simulink model "teleoperation_simscape"  (R2018a)
settings: Solver=ode45  StartTime=0.0  StopTime=10  RelTol=1e-3
values from neighbouring files (symbols this model uses):
  B_e = 0.01    [simulinkTeleop.m]
  B_h = humanDamp*armL    (= 0.4)    [simulinkTeleop.m]
  B_v = 0.15    [simulinkTeleop.m]
  J_m = 0.0005    [simulinkTeleop.m]
  J_s = 0.0005    [simulinkTeleop.m]
  J_v = 0.0    (= 0)    [simulinkTeleop.m]
  K_e = 1000    [simulinkTeleop.m]
  K_h = humanStiff*armL    (= 20)    [simulinkTeleop.m]
  K_v = 100.0    (= 100)    [simulinkTeleop.m]
  theta_s_contact = -0.0    (= 0)    [simulinkTeleop.m]
undefined symbols (not defined in the file or in its folder): X, Y, Z
libraries: sm_lib x14, cstblocks x5, nesl_utility x3, simulink x1
settings Model: Creator=dinies33  LastModifiedBy=giuseppe

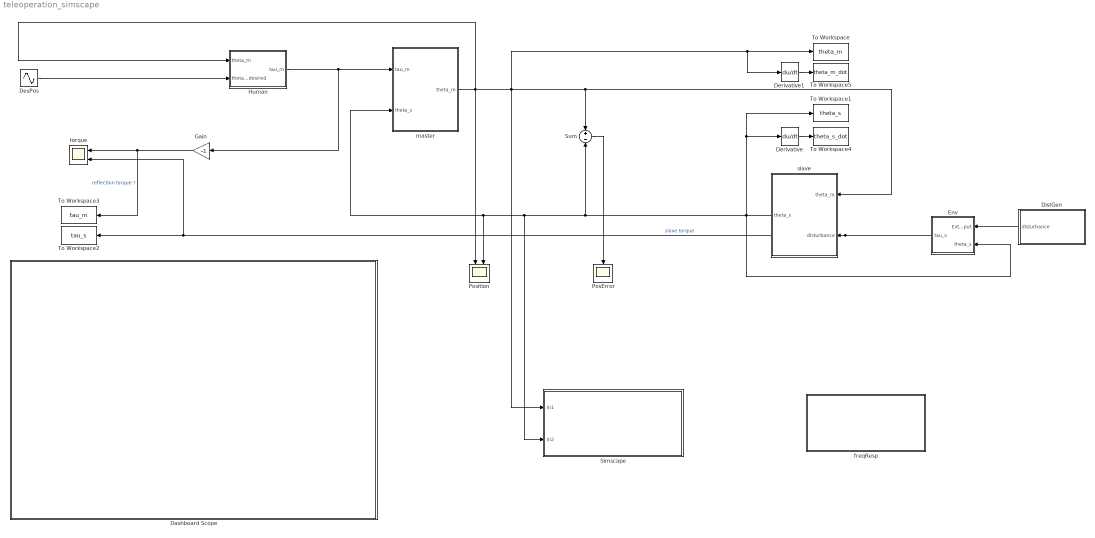
== system teleoperation_simscape ==
  Dashboard Scope : Subsystem  DialogController=hmiCreateDDGDialog  IsWebBlock=on  mask(MWDashboardBlock){webBlockId=d953983e-eab8-4310-ba24-9145e9f5b59c, webBlockType=sdiscope, ShowInitialText=on, HMISrcModelName=teleoperation_simscape}
      mask prompts: webBlockId "WebBlock Id"; webBlockType "WebBlock Type"; HMISrcModelName "Source Model"
      mask help: SimulinkHMI:dialogs:HMIScopeDialogDesc
      mask Help: helpview([docroot '/mapfiles/simulink.map'], 'hmi_scope')
      mask Display:
      | if strcmp(get_param(bdroot(gcb),'BlockDiagramType'), 'library')
      |     image([(matlabroot) '/toolbox/simulink/hmi/icons/DashboardScope.png']);
      | end
  Derivative : Derivative  CoefficientInTFapproximation=0
  Derivative1 : Derivative  CoefficientInTFapproximation=0
  DesPos : Sin  Amplitude=0.18  Frequency=0.11*(6.28)  SampleTime=0
  DistGen : Subsystem
  Env : Subsystem
  Gain : Gain  Gain=-1
  Human : Subsystem
  PosError : Scope
  Position : Scope  NumInputPorts=2
  Simscape : Subsystem
  Sum : Sum  Inputs=+-
  To Workspace : ToWorkspace  VariableName=theta_m  SampleTime=-1
  To Workspace1 : ToWorkspace  VariableName=theta_s  SampleTime=-1
  To Workspace2 : ToWorkspace  VariableName=tau_s  SampleTime=-1
  To Workspace3 : ToWorkspace  VariableName=tau_m  SampleTime=-1
  To Workspace4 : ToWorkspace  VariableName=theta_s_dot  SampleTime=-1
  To Workspace5 : ToWorkspace  VariableName=theta_m_dot  SampleTime=-1
  freqResp : Subsystem
  master : Subsystem
  "slave " : Subsystem
  torque : Scope  NumInputPorts=2
  wires:
  Env/1("tau_s ") -> torque/2, To Workspace2/1, "slave "/2(disturbance)  "slave torque"
  DesPos/1 -> Human/2(theta_desired)
  master/1(theta_m) -> Sum/1, "slave "/1("theta_m "), Derivative1/1, To Workspace/1, Simscape/1(In1), Human/1(theta_m), Position/1
  Human/1(tau_m) -> Gain/1, master/1(tau_m)
  "slave "/1(theta_s) -> Derivative/1, To Workspace1/1, Sum/2, Simscape/2(In2), master/2(theta_s), Position/2, Env/2(theta_s)
  Gain/1 -> To Workspace3/1, torque/1  "reflection torque ?"
  Sum/1 -> PosError/1
  Derivative1/1 -> To Workspace5/1
  Derivative/1 -> To Workspace4/1
  DistGen/1(disturbance) -> Env/1(External_input)

== system teleoperation_simscape/Dashboard Scope ==

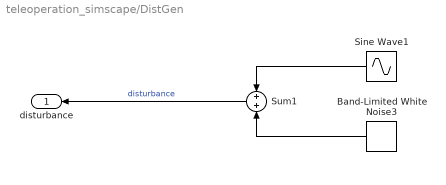
== system teleoperation_simscape/DistGen ==
  Band-Limited White Noise3 : simulink/Sources/Band-Limited White Noise  Cov=0.001  Ts=1/20  seed=[12345]
  Sine Wave1 : Sin  Amplitude=0.015  Frequency=20*(6.28)  SampleTime=0
  Sum1 : Sum
  disturbance : Outport
  wires:
  Band-Limited White Noise3/1 -> Sum1/2
  Sum1/1 -> disturbance/1  "disturbance"
  Sine Wave1/1 -> Sum1/1

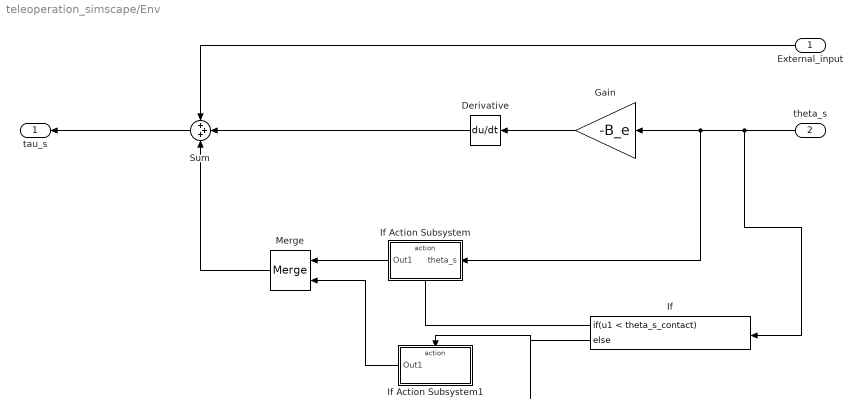
== system teleoperation_simscape/Env ==
  External_input : Inport
  theta_s : Inport  Port=2
  Derivative : Derivative  CoefficientInTFapproximation=0
  Gain : Gain  Gain=-B_e
  If : If  IfExpression=u1 < theta_s_contact
  If Action Subsystem : Subsystem  TreatAsAtomicUnit=on
  If Action Subsystem1 : Subsystem  TreatAsAtomicUnit=on
  Merge : Merge
  Sum : Sum  Inputs=+++
  "tau_s " : Outport
  wires:
  External_input/1 -> Sum/1
  theta_s/1 -> If/1, If Action Subsystem/1(theta_s), Gain/1
  Gain/1 -> Derivative/1
  Derivative/1 -> Sum/2
  Sum/1 -> "tau_s "/1
  If/2 -> If Action Subsystem1/Action
  If/1 -> If Action Subsystem/Action
  If Action Subsystem1/1(Out1) -> Merge/2
  If Action Subsystem/1(Out1) -> Merge/1
  Merge/1 -> Sum/3

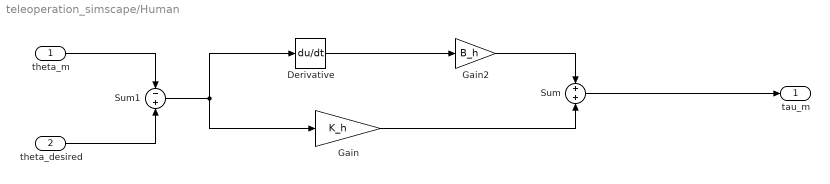
== system teleoperation_simscape/Human ==
  theta_m : Inport
  theta_desired : Inport  Port=2
  Derivative : Derivative  CoefficientInTFapproximation=0
  Gain : Gain  Gain=K_h
  Gain2 : Gain  Gain=B_h
  Sum : Sum  Inputs=+|+
  Sum1 : Sum  Inputs=-|+
  tau_m : Outport
  wires:
  Derivative/1 -> Gain2/1
  theta_m/1 -> Sum1/1
  theta_desired/1 -> Sum1/2
  Sum1/1 -> Derivative/1, Gain/1
  Gain2/1 -> Sum/1
  Gain/1 -> Sum/2
  Sum/1 -> tau_m/1

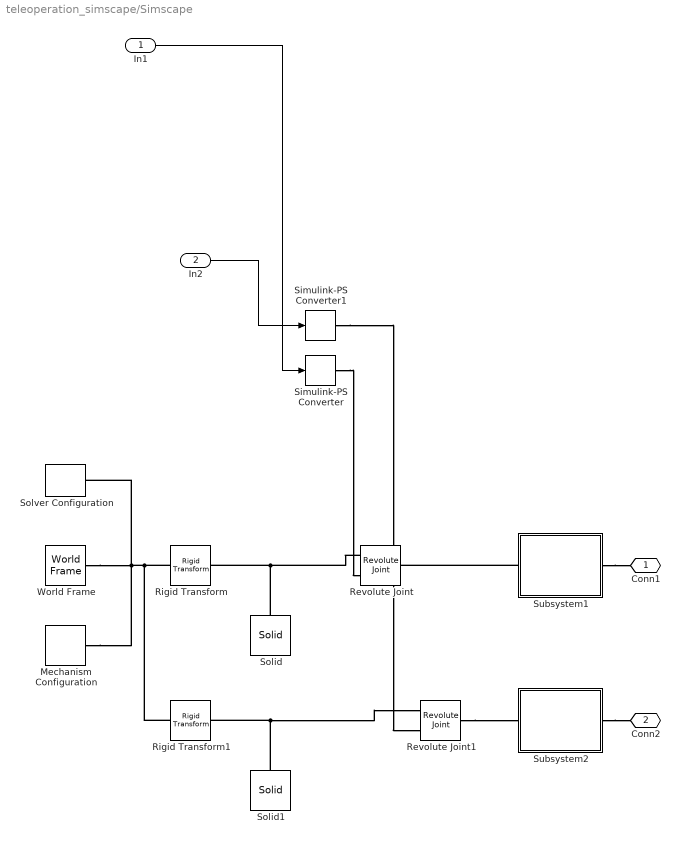
== system teleoperation_simscape/Simscape ==
  In1 : Inport
  In2 : Inport  Port=2
  Mechanism Configuration : sm_lib/Utilities/Mechanism Configuration  UniformGravity=Constant  GravityVector=[0 -9.81 0]  GravityUnits=m/s^2  LinearizationDelta=0.001
  Revolute Joint : sm_lib/Joints/Revolute Joint  SenseConstraintForce=off  SenseConstraintForceX=off  SenseConstraintForceY=off  SenseConstraintForceZ=off  SenseConstraintTorque=off  SenseConstraintTorqueX=off  SenseConstraintTorqueY=off  SenseConstraintTorqueZ=off  SenseTotalForce=off  SenseTotalForceX=off  SenseTotalForceY=off  SenseTotalForceZ=off  SenseTotalTorque=off  SenseTotalTorqueX=off  SenseTotalTorqueY=off  SenseTotalTorqueZ=off  CompositeWrenchDir=FollowerOnBase  CompositeWrenchFrame=BaseFrame  EquilibriumPosition=0  EquilibriumPositionUnits=deg  SpringStiffness=0  SpringStiffnessUnits=N*m/deg  DampingCoefficient=0  DampingCoefficientUnits=N*m/(deg/s)  TorqueActuationMode=ComputedTorque  MotionActuationMode=InputMotion  SensePosition=off  SenseVelocity=off  SenseAcceleration=off  SenseTorqueForce=off  PositionTargetSpecify=off  PositionTargetPriority=High  PositionTargetValue=0  PositionTargetValueUnits=deg  VelocityTargetSpecify=off  VelocityTargetPriority=High  VelocityTargetValue=0  VelocityTargetValueUnits=deg/s
  Revolute Joint1 : sm_lib/Joints/Revolute Joint  SenseConstraintForce=off  SenseConstraintForceX=off  SenseConstraintForceY=off  SenseConstraintForceZ=off  SenseConstraintTorque=off  SenseConstraintTorqueX=off  SenseConstraintTorqueY=off  SenseConstraintTorqueZ=off  SenseTotalForce=off  SenseTotalForceX=off  SenseTotalForceY=off  SenseTotalForceZ=off  SenseTotalTorque=off  SenseTotalTorqueX=off  SenseTotalTorqueY=off  SenseTotalTorqueZ=off  CompositeWrenchDir=FollowerOnBase  CompositeWrenchFrame=BaseFrame  EquilibriumPosition=0  EquilibriumPositionUnits=deg  SpringStiffness=0  SpringStiffnessUnits=N*m/deg  DampingCoefficient=0  DampingCoefficientUnits=N*m/(deg/s)  TorqueActuationMode=ComputedTorque  MotionActuationMode=InputMotion  SensePosition=off  SenseVelocity=off  SenseAcceleration=off  SenseTorqueForce=off  PositionTargetSpecify=off  PositionTargetPriority=High  PositionTargetValue=0  PositionTargetValueUnits=deg  VelocityTargetSpecify=off  VelocityTargetPriority=High  VelocityTargetValue=0  VelocityTargetValueUnits=deg/s
  Rigid Transform : sm_lib/Frames and Transforms/Rigid Transform  TranslationMethod=StandardAxis  TranslationStandardOffset=-0.2  TranslationLengthUnit=m  TranslationStandardAxis=+X  TranslationCartesianOffset=[0 0 0]  TranslationROffset=0  TranslationROffsetUnits=m  TranslationZOffset=0  TranslationZOffsetUnits=m  TranslationThetaOffset=0  TranslationThetaOffsetUnits=deg  RotationMethod=StandardAxis  RotationAngleUnits=deg  RotationStandardAxis=+Z  RotationAngle=-90  RotationArbitraryAxis=[0 0 1]  FollAlignAxisA=+X  BaseAlignAxisA=+Y  FollAlignAxisB=+Y  BaseAlignAxisB=+Z  RotationSequenceAxes=FollowerAxes  RotationSequence=XYX  RotationSequenceAngles=[0 0 0]  RotationSequenceAnglesUnits=deg  RotationMatrix=[1 0 0; 0 1 0; 0 0 1]
  Rigid Transform1 : sm_lib/Frames and Transforms/Rigid Transform  TranslationMethod=StandardAxis  TranslationStandardOffset=0.2  TranslationLengthUnit=m  TranslationStandardAxis=+X  TranslationCartesianOffset=[0 0 0]  TranslationROffset=0  TranslationROffsetUnits=m  TranslationZOffset=0  TranslationZOffsetUnits=m  TranslationThetaOffset=0  TranslationThetaOffsetUnits=deg  RotationMethod=StandardAxis  RotationAngleUnits=deg  RotationStandardAxis=+Z  RotationAngle=-90  RotationArbitraryAxis=[0 0 1]  FollAlignAxisA=+X  BaseAlignAxisA=+Y  FollAlignAxisB=+Y  BaseAlignAxisB=+Z  RotationSequenceAxes=FollowerAxes  RotationSequence=XYX  RotationSequenceAngles=[0 0 0]  RotationSequenceAnglesUnits=deg  RotationMatrix=[1 0 0; 0 1 0; 0 0 1]
  Simulink-PS Converter : nesl_utility/Simulink-PS Converter  PhysicalDomain=network_engine_domain  SubClassName=ps_input  LeftPortType=input  RightPortType=output  PseudoPeriodic=off  Frequencies=[]  NoiseDistribution=none  NoiseParameters=[]  Unit=rad  AffineConversion=on  FilteringAndDerivatives=filter  SimscapeFilterOrder=2  InputFilterTimeConstant=0.001  UdotUserProvided=0
  Simulink-PS Converter1 : nesl_utility/Simulink-PS Converter  PhysicalDomain=network_engine_domain  SubClassName=ps_input  LeftPortType=input  RightPortType=output  PseudoPeriodic=off  Frequencies=[]  NoiseDistribution=none  NoiseParameters=[]  Unit=rad  AffineConversion=on  FilteringAndDerivatives=filter  SimscapeFilterOrder=2  InputFilterTimeConstant=0.001  UdotUserProvided=0
  Solid : sm_lib/Body Elements/Solid  InertiaType=CalculateFromGeometry  Mass=1  MassUnits=kg  CenterOfMass=[0 0 0]  CenterOfMassUnits=m  MomentsOfInertia=[1 1 1]  MomentsOfInertiaUnits=kg*m^2  ProductsOfInertia=[0 0 0]  ProductsOfInertiaUnits=kg*m^2  DensityBased=on  Density=1000  DensityUnits=kg/m^3  DoExposeReferenceFrame=on  SerializedFrames=<Frames/>  GraphicType=FromGeometry  MarkerShape=Sphere  MarkerSize=10  GraphicVisPropType=SimpleVisualProperties  GraphicDiffuseColor=[0.5 0.5 0.5]  GraphicSpecularColor=[0.5 0.5 0.5 1.0]  GraphicAmbientColor=[0.15 0.15 0.15 1.0]  GraphicEmissiveColor=[0.0 0.0 0.0 1.0]  GraphicShininess=75  GraphicOpacity=1.0  GeometryShape=Sphere  RectangleSize=[1 1]  RectangleSizeUnits=m  BrickDimensions=[1 1 1]  BrickDimensionUnits=cm  CylinderRadius=1  CylinderRadiusUnits=m  CylinderLength=1  CylinderLengthUnits=m  SphereRadius=0.01  SphereRadiusUnits=m  EllipsoidRadii=[1 1 1]  EllipsoidRadiiUnits=m  ExtrusionCrossSection=[1 1; -1 1; -1 -1; 1 -1]  ExtrusionCrossSectionUnits=m  ExtrusionLength=1  ExtrusionLengthUnits=m  PolygonNumSides=3  PolygonOuterRadius=1  PolygonOuterRadiusUnits=m  ExtGeomFileType=STEP  ExtGeomFileUnits=m  RevolutionCrossSection=[1 1; 1 -1; 2 -1; 2 1]  RevolutionCrossSectionUnits=m  RevolutionExtent=Full  RevolutionAngle=180  RevolutionAngleUnits=deg
  Solid1 : sm_lib/Body Elements/Solid  InertiaType=CalculateFromGeometry  Mass=1  MassUnits=kg  CenterOfMass=[0 0 0]  CenterOfMassUnits=m  MomentsOfInertia=[1 1 1]  MomentsOfInertiaUnits=kg*m^2  ProductsOfInertia=[0 0 0]  ProductsOfInertiaUnits=kg*m^2  DensityBased=on  Density=1000  DensityUnits=kg/m^3  DoExposeReferenceFrame=on  SerializedFrames=<Frames/>  GraphicType=FromGeometry  MarkerShape=Sphere  MarkerSize=10  GraphicVisPropType=SimpleVisualProperties  GraphicDiffuseColor=[0.5 0.5 0.5]  GraphicSpecularColor=[0.5 0.5 0.5 1.0]  GraphicAmbientColor=[0.15 0.15 0.15 1.0]  GraphicEmissiveColor=[0.0 0.0 0.0 1.0]  GraphicShininess=75  GraphicOpacity=1.0  GeometryShape=Sphere  RectangleSize=[1 1]  RectangleSizeUnits=m  BrickDimensions=[1 1 1]  BrickDimensionUnits=cm  CylinderRadius=1  CylinderRadiusUnits=m  CylinderLength=1  CylinderLengthUnits=m  SphereRadius=0.01  SphereRadiusUnits=m  EllipsoidRadii=[1 1 1]  EllipsoidRadiiUnits=m  ExtrusionCrossSection=[1 1; -1 1; -1 -1; 1 -1]  ExtrusionCrossSectionUnits=m  ExtrusionLength=1  ExtrusionLengthUnits=m  PolygonNumSides=3  PolygonOuterRadius=1  PolygonOuterRadiusUnits=m  ExtGeomFileType=STEP  ExtGeomFileUnits=m  RevolutionCrossSection=[1 1; 1 -1; 2 -1; 2 1]  RevolutionCrossSectionUnits=m  RevolutionExtent=Full  RevolutionAngle=180  RevolutionAngleUnits=deg
  Solver Configuration : nesl_utility/Solver Configuration  PhysicalDomain=network_engine_domain  SubClassName=solver  LeftPortType=input  RightPortType=generic  Tones=[]  Harmonics=[]  SimulateNoise=off  Profile=off  UseLocalSampling=off  EnableSwitchedLinearOptims=on  FrequencyDomain=off  UseCCode=off  RelTol=0.001  AbsTol=1e-06  MinStep=1e-09  ToWorkspace=off  RevertToSquareIcSolve=off  NumHomotopyIterations=100  PhasorMode=off  PhasorModeNumHarmonics=1  DoDC=off  ResidualTolerance=1e-09  UseLocalSolver=off  LocalSolverChoice=NE_BACKWARD_EULER_ADVANCER  LocalSolverSampleTime=0.001  DoFixedCost=off  MaxNonlinIter=3  MaxModeIter=2  LinearAlgebra=Sparse  EquationFormulation=NE_TIME_EF  DelaysMemoryBudget=1024  AutomaticFiltering=on  FilteringTimeConstant=0.001
  Subsystem1 : Subsystem  mask{L=0.1, r=0.01, rho=2700}
      mask prompts: L "Lenght (m)"; r "Radius (m)"; rho "Density (kg/m^3)"
  Subsystem2 : Subsystem  mask{L=0.1, r=0.01, rho=2700}
      mask prompts: L "Lenght (m)"; r "Radius (m)"; rho "Density (kg/m^3)"
  World Frame : sm_lib/Frames and Transforms/World Frame
  Conn1 : PMIOPort  Side=Right
  Conn2 : PMIOPort  Port=2  Side=Right
  wires:
  In1/1 -> Simulink-PS Converter/1
  In2/1 -> Simulink-PS Converter1/1
  connections:
  Simulink-PS Converter/RConn1 -- Revolute Joint/LConn2
  Subsystem1/LConn1 -- Revolute Joint/RConn1
  Subsystem2/RConn1 -- Conn2/RConn1
  Subsystem1/RConn1 -- Conn1/RConn1
  Solver Configuration/RConn1 -- Rigid Transform1/LConn1 -- Rigid Transform/LConn1 -- World Frame/RConn1 -- Mechanism Configuration/RConn1
  Simulink-PS Converter1/RConn1 -- Revolute Joint1/LConn2
  Revolute Joint1/RConn1 -- Subsystem2/LConn1
  Revolute Joint/LConn1 -- Solid/RConn1 -- Rigid Transform/RConn1
  Rigid Transform1/RConn1 -- Revolute Joint1/LConn1 -- Solid1/RConn1

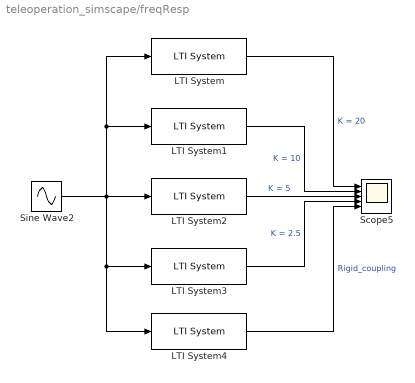
== system teleoperation_simscape/freqResp ==
  LTI System : cstblocks/LTI System  sys=set_1  IC=[]
  LTI System1 : cstblocks/LTI System  sys=set_2  IC=[]
  LTI System2 : cstblocks/LTI System  sys=set_3  IC=[]
  LTI System3 : cstblocks/LTI System  sys=set_4  IC=[]
  LTI System4 : cstblocks/LTI System  sys=rigid  IC=[]
  Scope5 : Scope  NumInputPorts=5
  Sine Wave2 : Sin  Amplitude=0.1  Frequency=10*(6.28)  SampleTime=0
  wires:
  LTI System1/1 -> Scope5/2  "K = 10"
  Sine Wave2/1 -> LTI System4/1, LTI System3/1, LTI System2/1, LTI System1/1, LTI System/1
  LTI System/1 -> Scope5/1  "K = 20"
  LTI System2/1 -> Scope5/3  "K = 5"
  LTI System4/1 -> Scope5/5  "Rigid_coupling"
  LTI System3/1 -> Scope5/4  "K = 2.5"

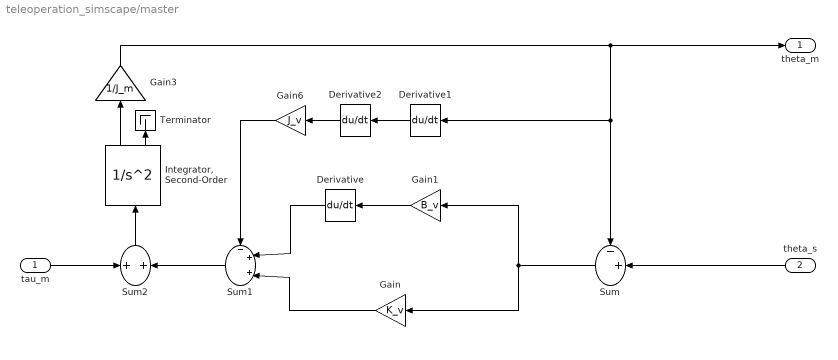
== system teleoperation_simscape/master ==
  tau_m : Inport
  theta_s : Inport  Port=2
  Derivative : Derivative  CoefficientInTFapproximation=0
  Derivative1 : Derivative  CoefficientInTFapproximation=0
  Derivative2 : Derivative  CoefficientInTFapproximation=0
  Gain : Gain  Gain=K_v
  Gain1 : Gain  Gain=B_v
  Gain3 : Gain  Gain=1/J_m
  Gain6 : Gain  Gain=J_v
  "Integrator, Second-Order" : SecondOrderIntegrator  ICX=0
  Sum : Sum  Inputs=-+|
  Sum1 : Sum  Inputs=-++|
  Sum2 : Sum  Inputs=+|+
  Terminator : Terminator
  theta_m : Outport
  wires:
  Derivative1/1 -> Derivative2/1
  "Integrator, Second-Order"/1 -> Gain3/1
  theta_s/1 -> Sum/2
  Gain/1 -> Sum1/3
  Sum/1 -> Gain/1, Gain1/1
  Sum1/1 -> Sum2/2
  Derivative2/1 -> Gain6/1
  Derivative/1 -> Sum1/2
  Gain6/1 -> Sum1/1
  Gain1/1 -> Derivative/1
  Sum2/1 -> "Integrator, Second-Order"/1
  tau_m/1 -> Sum2/1
  Gain3/1 -> theta_m/1, Derivative1/1, Sum/1
  "Integrator, Second-Order"/2 -> Terminator/1

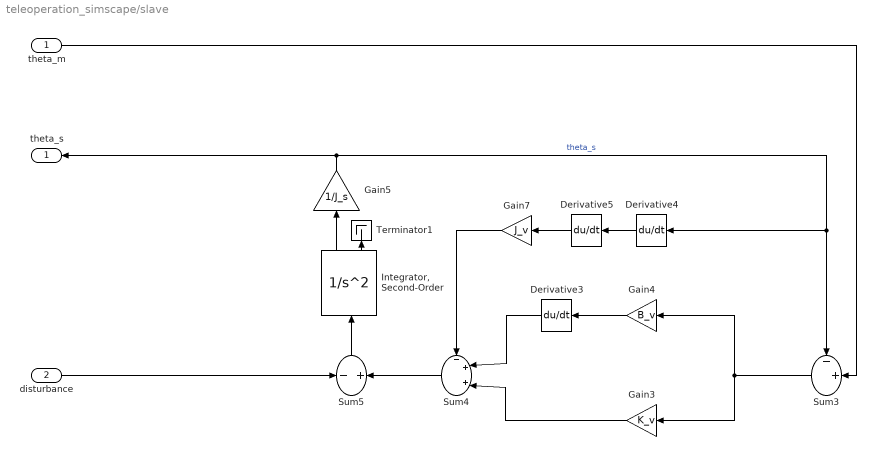
== system teleoperation_simscape/slave  ==
  "theta_m " : Inport
  disturbance : Inport  Port=2
  Derivative3 : Derivative  CoefficientInTFapproximation=0
  Derivative4 : Derivative  CoefficientInTFapproximation=0
  Derivative5 : Derivative  CoefficientInTFapproximation=0
  Gain3 : Gain  Gain=K_v
  Gain4 : Gain  Gain=B_v
  Gain5 : Gain  Gain=1/J_s
  Gain7 : Gain  Gain=J_v
  "Integrator, Second-Order" : SecondOrderIntegrator  ICX=0
  Sum3 : Sum  Inputs=-+|
  Sum4 : Sum  Inputs=-++|
  Sum5 : Sum  Inputs=-|+
  Terminator1 : Terminator
  theta_s : Outport
  wires:
  Sum5/1 -> "Integrator, Second-Order"/1
  Gain7/1 -> Sum4/1
  "Integrator, Second-Order"/1 -> Gain5/1
  Derivative5/1 -> Gain7/1
  Sum4/1 -> Sum5/2
  Derivative3/1 -> Sum4/2
  Gain4/1 -> Derivative3/1
  Gain5/1 -> Derivative4/1, Sum3/1, theta_s/1  "theta_s"
  Gain3/1 -> Sum4/3
  "theta_m "/1 -> Sum3/2
  Sum3/1 -> Gain3/1, Gain4/1
  Derivative4/1 -> Derivative5/1
  disturbance/1 -> Sum5/1
  "Integrator, Second-Order"/2 -> Terminator1/1

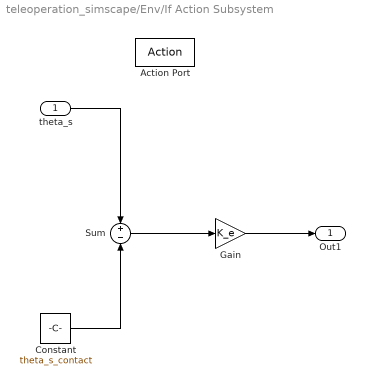
== system teleoperation_simscape/Env/If Action Subsystem ==
  theta_s : Inport
  Action Port : ActionPort  ActionType=then
  Constant : Constant  Value=theta_s_contact
  Gain : Gain  Gain=K_e
  Sum : Sum  Inputs=+-
  Out1 : Outport
  wires:
  theta_s/1 -> Sum/1
  Constant/1 -> Sum/2
  Sum/1 -> Gain/1
  Gain/1 -> Out1/1

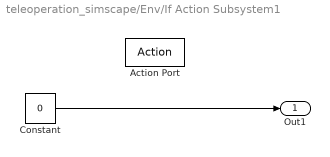
== system teleoperation_simscape/Env/If Action Subsystem1 ==
  Action Port : ActionPort  ActionType=else
  Constant : Constant  Value=0
  Out1 : Outport
  wires:
  Constant/1 -> Out1/1

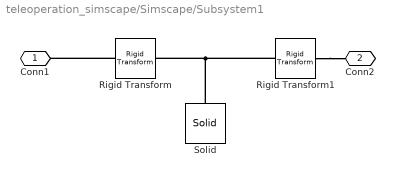
== system teleoperation_simscape/Simscape/Subsystem1 ==
  Rigid Transform : sm_lib/Frames and Transforms/Rigid Transform  TranslationMethod=StandardAxis  TranslationStandardOffset=L/2  TranslationLengthUnit=m  TranslationStandardAxis=-X  TranslationCartesianOffset=[0 0 0]  TranslationROffset=0  TranslationROffsetUnits=m  TranslationZOffset=0  TranslationZOffsetUnits=m  TranslationThetaOffset=0  TranslationThetaOffsetUnits=deg  RotationMethod=StandardAxis  RotationAngleUnits=deg  RotationStandardAxis=+Y  RotationAngle=90  RotationArbitraryAxis=[0 0 1]  FollAlignAxisA=+X  BaseAlignAxisA=+Y  FollAlignAxisB=+Y  BaseAlignAxisB=+Z  RotationSequenceAxes=FollowerAxes  RotationSequence=XYX  RotationSequenceAngles=[0 0 0]  RotationSequenceAnglesUnits=deg  RotationMatrix=[1 0 0; 0 1 0; 0 0 1]
  Rigid Transform1 : sm_lib/Frames and Transforms/Rigid Transform  TranslationMethod=StandardAxis  TranslationStandardOffset=L/2  TranslationLengthUnit=m  TranslationStandardAxis=+X  TranslationCartesianOffset=[0 0 0]  TranslationROffset=0  TranslationROffsetUnits=m  TranslationZOffset=0  TranslationZOffsetUnits=m  TranslationThetaOffset=0  TranslationThetaOffsetUnits=deg  RotationMethod=None  RotationAngleUnits=deg  RotationStandardAxis=+Z  RotationAngle=0.0  RotationArbitraryAxis=[0 0 1]  FollAlignAxisA=+X  BaseAlignAxisA=+Y  FollAlignAxisB=+Y  BaseAlignAxisB=+Z  RotationSequenceAxes=FollowerAxes  RotationSequence=XYX  RotationSequenceAngles=[0 0 0]  RotationSequenceAnglesUnits=deg  RotationMatrix=[1 0 0; 0 1 0; 0 0 1]
  Solid : sm_lib/Body Elements/Solid  InertiaType=CalculateFromGeometry  Mass=1  MassUnits=kg  CenterOfMass=[0 0 0]  CenterOfMassUnits=m  MomentsOfInertia=[1 1 1]  MomentsOfInertiaUnits=kg*m^2  ProductsOfInertia=[0 0 0]  ProductsOfInertiaUnits=kg*m^2  DensityBased=on  Density=rho  DensityUnits=kg/m^3  DoExposeReferenceFrame=on  SerializedFrames=<Frames/>  GraphicType=FromGeometry  MarkerShape=Sphere  MarkerSize=10  GraphicVisPropType=SimpleVisualProperties  GraphicDiffuseColor=[0.5 0.5 0.5]  GraphicSpecularColor=[0.5 0.5 0.5 1.0]  GraphicAmbientColor=[0.15 0.15 0.15 1.0]  GraphicEmissiveColor=[0.0 0.0 0.0 1.0]  GraphicShininess=75  GraphicOpacity=1.0  GeometryShape=Cylinder  RectangleSize=[1 1]  RectangleSizeUnits=m  BrickDimensions=[1 1 1]  BrickDimensionUnits=m  CylinderRadius=r  CylinderRadiusUnits=m  CylinderLength=L  CylinderLengthUnits=m  SphereRadius=1  SphereRadiusUnits=m  EllipsoidRadii=[1 1 1]  EllipsoidRadiiUnits=m  ExtrusionCrossSection=[1 1; -1 1; -1 -1; 1 -1]  ExtrusionCrossSectionUnits=m  ExtrusionLength=1  ExtrusionLengthUnits=m  PolygonNumSides=3  PolygonOuterRadius=1  PolygonOuterRadiusUnits=m  ExtGeomFileType=STEP  ExtGeomFileUnits=m  RevolutionCrossSection=[1 1; 1 -1; 2 -1; 2 1]  RevolutionCrossSectionUnits=m  RevolutionExtent=Full  RevolutionAngle=180  RevolutionAngleUnits=deg
  Conn1 : PMIOPort  Side=Left
  Conn2 : PMIOPort  Port=2  Side=Right
  connections:
  Rigid Transform1/LConn1 -- Rigid Transform/RConn1 -- Solid/RConn1
  Rigid Transform/LConn1 -- Conn1/RConn1
  Rigid Transform1/RConn1 -- Conn2/RConn1

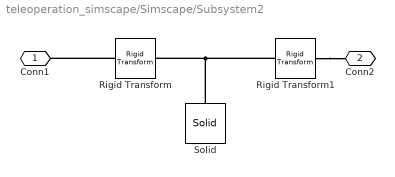
== system teleoperation_simscape/Simscape/Subsystem2 ==
  Rigid Transform : sm_lib/Frames and Transforms/Rigid Transform  TranslationMethod=StandardAxis  TranslationStandardOffset=L/2  TranslationLengthUnit=m  TranslationStandardAxis=-X  TranslationCartesianOffset=[0 0 0]  TranslationROffset=0  TranslationROffsetUnits=m  TranslationZOffset=0  TranslationZOffsetUnits=m  TranslationThetaOffset=0  TranslationThetaOffsetUnits=deg  RotationMethod=StandardAxis  RotationAngleUnits=deg  RotationStandardAxis=+Y  RotationAngle=90  RotationArbitraryAxis=[0 0 1]  FollAlignAxisA=+X  BaseAlignAxisA=+Y  FollAlignAxisB=+Y  BaseAlignAxisB=+Z  RotationSequenceAxes=FollowerAxes  RotationSequence=XYX  RotationSequenceAngles=[0 0 0]  RotationSequenceAnglesUnits=deg  RotationMatrix=[1 0 0; 0 1 0; 0 0 1]
  Rigid Transform1 : sm_lib/Frames and Transforms/Rigid Transform  TranslationMethod=StandardAxis  TranslationStandardOffset=L/2  TranslationLengthUnit=m  TranslationStandardAxis=+X  TranslationCartesianOffset=[0 0 0]  TranslationROffset=0  TranslationROffsetUnits=m  TranslationZOffset=0  TranslationZOffsetUnits=m  TranslationThetaOffset=0  TranslationThetaOffsetUnits=deg  RotationMethod=None  RotationAngleUnits=deg  RotationStandardAxis=+Z  RotationAngle=0.0  RotationArbitraryAxis=[0 0 1]  FollAlignAxisA=+X  BaseAlignAxisA=+Y  FollAlignAxisB=+Y  BaseAlignAxisB=+Z  RotationSequenceAxes=FollowerAxes  RotationSequence=XYX  RotationSequenceAngles=[0 0 0]  RotationSequenceAnglesUnits=deg  RotationMatrix=[1 0 0; 0 1 0; 0 0 1]
  Solid : sm_lib/Body Elements/Solid  InertiaType=CalculateFromGeometry  Mass=1  MassUnits=kg  CenterOfMass=[0 0 0]  CenterOfMassUnits=m  MomentsOfInertia=[1 1 1]  MomentsOfInertiaUnits=kg*m^2  ProductsOfInertia=[0 0 0]  ProductsOfInertiaUnits=kg*m^2  DensityBased=on  Density=rho  DensityUnits=kg/m^3  DoExposeReferenceFrame=on  SerializedFrames=<Frames/>  GraphicType=FromGeometry  MarkerShape=Sphere  MarkerSize=10  GraphicVisPropType=SimpleVisualProperties  GraphicDiffuseColor=[0.5 0.5 0.5]  GraphicSpecularColor=[0.5 0.5 0.5 1.0]  GraphicAmbientColor=[0.15 0.15 0.15 1.0]  GraphicEmissiveColor=[0.0 0.0 0.0 1.0]  GraphicShininess=75  GraphicOpacity=1.0  GeometryShape=Cylinder  RectangleSize=[1 1]  RectangleSizeUnits=m  BrickDimensions=[1 1 1]  BrickDimensionUnits=m  CylinderRadius=r  CylinderRadiusUnits=m  CylinderLength=L  CylinderLengthUnits=m  SphereRadius=1  SphereRadiusUnits=m  EllipsoidRadii=[1 1 1]  EllipsoidRadiiUnits=m  ExtrusionCrossSection=[1 1; -1 1; -1 -1; 1 -1]  ExtrusionCrossSectionUnits=m  ExtrusionLength=1  ExtrusionLengthUnits=m  PolygonNumSides=3  PolygonOuterRadius=1  PolygonOuterRadiusUnits=m  ExtGeomFileType=STEP  ExtGeomFileUnits=m  RevolutionCrossSection=[1 1; 1 -1; 2 -1; 2 1]  RevolutionCrossSectionUnits=m  RevolutionExtent=Full  RevolutionAngle=180  RevolutionAngleUnits=deg
  Conn1 : PMIOPort  Side=Left
  Conn2 : PMIOPort  Port=2  Side=Right
  connections:
  Rigid Transform1/RConn1 -- Conn2/RConn1
  Rigid Transform/LConn1 -- Conn1/RConn1
  Solid/RConn1 -- Rigid Transform/RConn1 -- Rigid Transform1/LConn1
